simulink model "GNC2026W"  (R2024b)
settings: Solver=ode4  StartTime=0.0  StopTime=tsim  FixedStep=baseRate
values from neighbouring files (symbols this model uses):
  a = 1    [Run_Initializer.m]    (also in UKFoptimization.m)
  a1 = 0.236940    (= 0.23694)    [DrawARM.m]    (also in Run_Initializer.m = 2)
  a2 = 0.281536    [DrawARM.m]    (also in Run_Initializer.m = 2)
  a3 = 0.0621    [DrawARM.m]    (also in Run_Initializer.m = 2)
  A_c = eye(3)    [Run_Initializer.m]
  alpha = diag([a1; a2; a3])    [Run_Initializer.m]    (also in overlapping_trajectories.m = alpha_values1(ii); plotTrajectory.m = alpha_values(ii); plotfig.m = alpha_values(ii))
  b = 2    [Run_Initializer.m]    (also in UKFoptimization.m)
  b0 = 0.230400    (= 0.2304)    [DrawARM.m]
  b1 = 0.078980    (= 0.07898)    [DrawARM.m]
  b2 = 0.070384    [DrawARM.m]
  b3 = 0.070685    [DrawARM.m]
  CVrate = 1/5    (= 0.2)    [Run_Initializer.m]
  dt = baseRate    [Run_Initializer.m]    (also in UKFoptimization.m = 0.05; rms_plots.m = median(diff(tA)))
  F_u = zeros(3,1)    [Run_Initializer.m]
  fNum = 1    [Run_Initializer.m]
  gamma = r - (excess + shrink + bracketwidth)    (= 0.05023)    [DrawSpacecraft.m]    (also in Run_Initializer.m = diag([g1; g2; g3]))
  Gamma1_el = 0.12    [Run_Initializer.m]
  Gamma1_sh = 0.005    [Run_Initializer.m]
  Gamma1_wr = 0.025    [Run_Initializer.m]
  Gamma2_el = 5    [Run_Initializer.m]
  Gamma2_sh = 5    [Run_Initializer.m]
  Gamma2_wr = 5    [Run_Initializer.m]
  Gamma3_el = 10    [Run_Initializer.m]
  Gamma3_sh = 40    [Run_Initializer.m]
  Gamma3_wr = 40    [Run_Initializer.m]
  Gamma4_el = 0.039    [Run_Initializer.m]
  Gamma4_sh = 0.015    [Run_Initializer.m]
  Gamma4_wr = 0.029    [Run_Initializer.m]
  Gamma5_el = 800    [Run_Initializer.m]
  Gamma5_sh = 800    [Run_Initializer.m]
  Gamma5_wr = 800    [Run_Initializer.m]
  Gamma6_el = 0.000001    (= 1e-06)    [Run_Initializer.m]
  Gamma6_sh = 0.005    [Run_Initializer.m]
  Gamma6_wr = 0.02    [Run_Initializer.m]
  k = 5    [Run_Initializer.m]    (also in UKFoptimization.m)
  Kd_elarm = 0.8    [Run_Initializer.m]
  Kd_sharm = 1.0    (= 1)    [Run_Initializer.m]
  Kd_wrarm = 0.6    [Run_Initializer.m]
  Kp_elarm = 1.2    [Run_Initializer.m]
  Kp_sharm = 1.5    [Run_Initializer.m]
  Kp_wrarm = 1.0    (= 1)    [Run_Initializer.m]
  Mc_inv = inv(M_c)    [Run_Initializer.m]
  Phi = 73.2749*pi/180    (= 1.27888826407)    [DrawARM.m]
  PWMFreq = 5    [Run_Initializer.m]
  R = [cos(theta) -sin(theta) ... (first row only)    [Run_Initializer.m]    (also in UKFoptimization.m = diag([rx, rx, rt]))
  sep1 = 0.60    (= 0.6)    [Run_Initializer.m]
  sep2 = 0.30    (= 0.3)    [Run_Initializer.m]
  sep3 = 0.30    (= 0.3)    [Run_Initializer.m]
  Tz_lim_elarm = .1    (= 0.1)    [Run_Initializer.m]
  Tz_lim_sharm = .1    (= 0.1)    [Run_Initializer.m]
  Tz_lim_wrarm = .1    (= 0.1)    [Run_Initializer.m]
  VISinLoop = 1    [Run_Initializer.m]
  X1_blk = 0.4    [Run_Initializer.m]
  X2_blk = 0.4    [Run_Initializer.m]
  X3_blk = 0.4    [Run_Initializer.m]
  Y1_blk = 0.4    [Run_Initializer.m]
  Y2_blk = 0.4    [Run_Initializer.m]
  Y3_blk = 0.4    [Run_Initializer.m]
undefined symbols (not defined in the file or in its folder): baseRate, dataRate, DiscIntNeverNeededParam, drop_states_ARM, drop_states_BLACK, drop_states_BLUE, drop_states_RED, F_red_X_nominal, F_red_Y_nominal, F_thrusters_BLACK, F_thrusters_BLUE, F_thrusters_RED, home_states_BLACK, home_states_BLUE, home_states_RED, IBLACK, IBLUE, IDIST, IEE, init_states_BLACK, init_states_BLUE, init_states_RED, IPROX, IRED, K_BLACK, K_BLUE, K_RED, Kd_tb, Kd_tblue, Kd_tr, Kd_xb, Kd_xblue, Kd_xr, Kd_yb, Kd_yblue, Kd_yr, Kp_tb, Kp_tblue, Kp_tr, Kp_xb, Kp_xblue, Kp_xr, Kp_yb, Kp_yblue, Kp_yr, mBLACK, mBLUE, mDIST, mEE, mPROX, mRED, Phase0_End, Phase1_End, Phase2_End, Phase3_End, Phase3_SubPhase1_End, Phase3_SubPhase2_End, Phase3_SubPhase3_End, Phase3_SubPhase4_End, Phase4_End ... (+10)
libraries: simulink x30, nvidiaSharedBlocks x20, MainLibrary x5, dspinverses x3, commrandsrc3 x1, nvidiaIMUSensorslib x1
(part 3 of 9)

== system GNC2026W/3 - Control/Default PD (ARM) ==
  Action Port : ActionPort  ActionPortLabel=if(u1 == 1 )
  Constant7 : Constant
  Data Store Read2 : DataStoreRead  DataStoreName=ARM_Path  IndexOptions=Index vector (dialog)  Indices=1  OutputSizes=1
  Data Store Read4 : DataStoreRead  DataStoreName=isSim  IndexOptions=Index vector (dialog)  Indices=1  OutputSizes=1
  Data Store Write12 : DataStoreWrite  DataStoreName=ARM_Control_Mode  IndexOptions=Index vector (dialog)  Indices=1  OutputSizes=1
  Demux : Demux  Outputs=3
  "If 'simMode' set to '1', then this is a simulation and the dynamics will be simulated. Otherwise, this is an experiment, and the simulation will not be run." : If  IfExpression=u1 == 1
  Merge3 : Merge
  Merge4 : Merge
  Merge5 : Merge
  Mux : Mux  Inputs=3
  Passthrough for Experiment : Subsystem  TreatAsAtomicUnit=on
  Scope : Scope
  Simulated Position Controller : Subsystem  TreatAsAtomicUnit=on
  u : Outport
  wires:
  Passthrough for Experiment/3(q3_command) -> Merge5/2
  Data Store Read4/1 -> "If 'simMode' set to '1', then this is a simulation and the dynamics will be simulated. Otherwise, this is an experiment, and the simulation will not be run."/1
  Demux/3 -> Passthrough for Experiment/3(q3_desired), Simulated Position Controller/3(q3_desired)
  Simulated Position Controller/1(q1_command) -> Merge3/1
  Simulated Position Controller/3(q3_command) -> Merge5/1
  "If 'simMode' set to '1', then this is a simulation and the dynamics will be simulated. Otherwise, this is an experiment, and the simulation will not be run."/1 -> Simulated Position Controller/Action
  Demux/2 -> Passthrough for Experiment/2(q2_desired), Simulated Position Controller/2(q2_desired)
  Passthrough for Experiment/2(q2_command) -> Merge4/2
  Simulated Position Controller/2(q2_command) -> Merge4/1
  Constant7/1 -> Data Store Write12/1
  Passthrough for Experiment/1(q1_command) -> Merge3/2
  Demux/1 -> Passthrough for Experiment/1(q1_desired), Simulated Position Controller/1(q1_desired)
  "If 'simMode' set to '1', then this is a simulation and the dynamics will be simulated. Otherwise, this is an experiment, and the simulation will not be run."/2 -> Passthrough for Experiment/Action
  Merge3/1 -> Mux/1
  Merge4/1 -> Mux/2
  Merge5/1 -> Mux/3
  Mux/1 -> Scope/1, u/1
  Data Store Read2/1 -> Demux/1

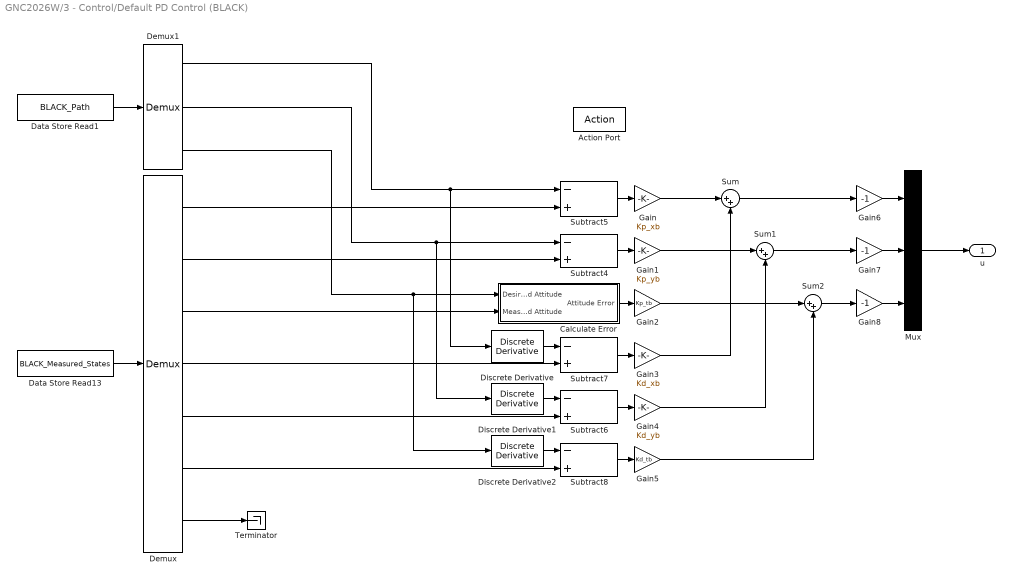
== system GNC2026W/3 - Control/Default PD Control (BLACK) ==
  Action Port : ActionPort  ActionPortLabel=if(u1 == 1 )
  Calculate Error : Subsystem
  Data Store Read1 : DataStoreRead  DataStoreName=BLACK_Path  IndexOptions=Index vector (dialog)  Indices=1  OutputSizes=1
  Data Store Read13 : DataStoreRead  DataStoreName=BLACK_Measured_States  IndexOptions=Index vector (dialog)  Indices=1  OutputSizes=1
  Demux : Demux  Outputs=[1,1,1,1,1,1,3]
  Demux1 : Demux  Outputs=3
  Discrete Derivative : simulink/Discrete/Discrete Derivative  gainval=1.0  ICPrevScaledInput=0.0  OutMin=[]  OutMax=[]  OutDataType=fixdt(1, 16)  OutScaling=2^-10  DoSatur=off
  Discrete Derivative1 : simulink/Discrete/Discrete Derivative  gainval=1.0  ICPrevScaledInput=0.0  OutMin=[]  OutMax=[]  OutDataType=fixdt(1, 16)  OutScaling=2^-10  DoSatur=off
  Discrete Derivative2 : simulink/Discrete/Discrete Derivative  gainval=1.0  ICPrevScaledInput=0.0  OutMin=[]  OutMax=[]  OutDataType=fixdt(1, 16)  OutScaling=2^-10  DoSatur=off
  Gain : Gain  Gain=Kp_xb
  Gain1 : Gain  Gain=Kp_yb
  Gain2 : Gain  Gain=Kp_tb
  Gain3 : Gain  Gain=Kd_xb
  Gain4 : Gain  Gain=Kd_yb
  Gain5 : Gain  Gain=Kd_tb
  Gain6 : Gain  Gain=-1
  Gain7 : Gain  Gain=-1
  Gain8 : Gain  Gain=-1
  Mux : Mux  Inputs=3
  Subtract{4..8} (5 alike) : Sum  Inputs=-+
  Sum : Sum  Inputs=|++
  Sum1 : Sum  Inputs=|++
  Sum2 : Sum  Inputs=|++
  Terminator : Terminator
  u : Outport
  wires:
  Demux/6 -> Subtract8/2
  Subtract8/1 -> Gain5/1
  Gain8/1 -> Mux/3
  Discrete Derivative2/1 -> Subtract8/1
  Gain1/1 -> Sum1/1
  Subtract5/1 -> Gain/1
  Discrete Derivative1/1 -> Subtract6/1
  Subtract6/1 -> Gain4/1
  Demux/2 -> Subtract4/2
  Demux/1 -> Subtract5/2
  Sum1/1 -> Gain7/1
  Demux/4 -> Subtract7/2
  Demux1/3 -> Calculate Error/1(Desired Attitude), Discrete Derivative2/1
  Sum/1 -> Gain6/1
  Subtract4/1 -> Gain1/1
  Demux/3 -> Calculate Error/2(Measured Attitude)
  Subtract7/1 -> Gain3/1
  Gain3/1 -> Sum/2
  Mux/1 -> u/1
  Gain4/1 -> Sum1/2
  Demux1/2 -> Discrete Derivative1/1, Subtract4/1
  Gain/1 -> Sum/1
  Demux/5 -> Subtract6/2
  Gain5/1 -> Sum2/2
  Discrete Derivative/1 -> Subtract7/1
  Demux1/1 -> Discrete Derivative/1, Subtract5/1
  Sum2/1 -> Gain8/1
  Calculate Error/1(Attitude Error) -> Gain2/1
  Gain7/1 -> Mux/2
  Gain6/1 -> Mux/1
  Gain2/1 -> Sum2/1
  Data Store Read13/1 -> Demux/1
  Demux/7 -> Terminator/1
  Data Store Read1/1 -> Demux1/1

== system GNC2026W/3 - Control/Default PD Control (BLUE) ==
  Action Port : ActionPort  ActionPortLabel=if(u1 == 1 )
  Calculate Error : Subsystem
  Data Store Read1 : DataStoreRead  DataStoreName=BLUE_Path  IndexOptions=Index vector (dialog)  Indices=1  OutputSizes=1
  Data Store Read2 : DataStoreRead  DataStoreName=BLUE_Measured_States  IndexOptions=Index vector (dialog)  Indices=1  OutputSizes=1
  Demux : Demux  Outputs=[1,1,1,1,1,1,3]
  Demux1 : Demux  Outputs=3
  Discrete Derivative : simulink/Discrete/Discrete Derivative  gainval=1.0  ICPrevScaledInput=0.0  OutMin=[]  OutMax=[]  OutDataType=fixdt(1, 16)  OutScaling=2^-10  DoSatur=off
  Discrete Derivative1 : simulink/Discrete/Discrete Derivative  gainval=1.0  ICPrevScaledInput=0.0  OutMin=[]  OutMax=[]  OutDataType=fixdt(1, 16)  OutScaling=2^-10  DoSatur=off
  Discrete Derivative2 : simulink/Discrete/Discrete Derivative  gainval=1.0  ICPrevScaledInput=0.0  OutMin=[]  OutMax=[]  OutDataType=fixdt(1, 16)  OutScaling=2^-10  DoSatur=off
  Gain : Gain  Gain=Kp_xblue
  Gain1 : Gain  Gain=Kp_yblue
  Gain2 : Gain  Gain=Kp_tblue
  Gain3 : Gain  Gain=Kd_xblue
  Gain4 : Gain  Gain=Kd_yblue
  Gain5 : Gain  Gain=Kd_tblue
  Gain6 : Gain  Gain=-1
  Gain7 : Gain  Gain=-1
  Gain8 : Gain  Gain=-1
  Mux3 : Mux  Inputs=3
  Subtract{4..8} (5 alike) : Sum  Inputs=-+
  Sum : Sum  Inputs=|++
  Sum1 : Sum  Inputs=|++
  Sum2 : Sum  Inputs=|++
  Terminator : Terminator
  u : Outport
  wires:
  Sum/1 -> Gain6/1
  Mux3/1 -> u/1
  Gain3/1 -> Sum/2
  Sum2/1 -> Gain8/1
  Gain5/1 -> Sum2/2
  Sum1/1 -> Gain7/1
  Gain6/1 -> Mux3/1
  Gain4/1 -> Sum1/2
  Gain1/1 -> Sum1/1
  Gain2/1 -> Sum2/1
  Gain8/1 -> Mux3/3
  Gain7/1 -> Mux3/2
  Gain/1 -> Sum/1
  Demux1/1 -> Discrete Derivative/1, Subtract5/1
  Discrete Derivative/1 -> Subtract7/1
  Demux1/3 -> Calculate Error/1(Desired Attitude), Discrete Derivative2/1
  Discrete Derivative1/1 -> Subtract6/1
  Demux/5 -> Subtract6/2
  Demux/3 -> Calculate Error/2(Measured Attitude)
  Demux/7 -> Terminator/1
  Data Store Read1/1 -> Demux1/1
  Demux/2 -> Subtract4/2
  Demux/1 -> Subtract5/2
  Demux/4 -> Subtract7/2
  Demux1/2 -> Discrete Derivative1/1, Subtract4/1
  Discrete Derivative2/1 -> Subtract8/1
  Data Store Read2/1 -> Demux/1
  Demux/6 -> Subtract8/2
  Subtract5/1 -> Gain/1
  Subtract4/1 -> Gain1/1
  Calculate Error/1(Attitude Error) -> Gain2/1
  Subtract7/1 -> Gain3/1
  Subtract6/1 -> Gain4/1
  Subtract8/1 -> Gain5/1

== system GNC2026W/3 - Control/Default PD Control (RED) ==
  Action Port : ActionPort  ActionPortLabel=if(u1 == 1 )
  Calculate Error : Subsystem
  Data Store Read1 : DataStoreRead  DataStoreName=RED_Path  IndexOptions=Index vector (dialog)  Indices=1  OutputSizes=1
  Data Store Read13 : DataStoreRead  DataStoreName=RED_Measured_States  IndexOptions=Index vector (dialog)  Indices=1  OutputSizes=1
  Demux : Demux  Outputs=[1,1,1,1,1,1,3]
  Demux1 : Demux  Outputs=3
  Discrete Derivative : simulink/Discrete/Discrete Derivative  gainval=1.0  ICPrevScaledInput=0.0  OutMin=[]  OutMax=[]  OutDataType=fixdt(1, 16)  OutScaling=2^-10  DoSatur=off
  Discrete Derivative1 : simulink/Discrete/Discrete Derivative  gainval=1.0  ICPrevScaledInput=0.0  OutMin=[]  OutMax=[]  OutDataType=fixdt(1, 16)  OutScaling=2^-10  DoSatur=off
  Discrete Derivative2 : simulink/Discrete/Discrete Derivative  gainval=1.0  ICPrevScaledInput=0.0  OutMin=[]  OutMax=[]  OutDataType=fixdt(1, 16)  OutScaling=2^-10  DoSatur=off
  Gain : Gain  Gain=Kp_xr
  Gain1 : Gain  Gain=Kp_yr
  Gain2 : Gain  Gain=Kp_tr
  Gain3 : Gain  Gain=Kd_xr
  Gain4 : Gain  Gain=Kd_yr
  Gain5 : Gain  Gain=Kd_tr
  Gain6 : Gain  Gain=-1
  Gain7 : Gain  Gain=-1
  Gain8 : Gain  Gain=-1
  Mux : Mux  Inputs=3
  Subtract{4..8} (5 alike) : Sum  Inputs=-+
  Sum : Sum  Inputs=|++
  Sum1 : Sum  Inputs=|++
  Sum2 : Sum  Inputs=|++
  Terminator : Terminator
  u1 : Outport
  wires:
  Gain6/1 -> Mux/1
  Gain8/1 -> Mux/3
  Gain1/1 -> Sum1/1
  Sum/1 -> Gain6/1
  Gain5/1 -> Sum2/2
  Gain3/1 -> Sum/2
  Sum1/1 -> Gain7/1
  Mux/1 -> u1/1
  Gain4/1 -> Sum1/2
  Sum2/1 -> Gain8/1
  Gain/1 -> Sum/1
  Gain7/1 -> Mux/2
  Gain2/1 -> Sum2/1
  Demux1/2 -> Discrete Derivative1/1, Subtract4/1
  Demux/2 -> Subtract4/2
  Demux1/3 -> Calculate Error/1(Desired Attitude), Discrete Derivative2/1
  Discrete Derivative1/1 -> Subtract6/1
  Demux/4 -> Subtract7/2
  Data Store Read13/1 -> Demux/1
  Demux/1 -> Subtract5/2
  Discrete Derivative/1 -> Subtract7/1
  Data Store Read1/1 -> Demux1/1
  Demux/5 -> Subtract6/2
  Demux/3 -> Calculate Error/2(Measured Attitude)
  Demux/7 -> Terminator/1
  Discrete Derivative2/1 -> Subtract8/1
  Demux1/1 -> Discrete Derivative/1, Subtract5/1
  Demux/6 -> Subtract8/2
  Subtract5/1 -> Gain/1
  Subtract4/1 -> Gain1/1
  Calculate Error/1(Attitude Error) -> Gain2/1
  Subtract7/1 -> Gain3/1
  Subtract6/1 -> Gain4/1
  Subtract8/1 -> Gain5/1

== system GNC2026W/3 - Control/Disable Control (ARM) ==
  Action Port : ActionPort  ActionPortLabel=else
  Constant7 : Constant  Value=0
  Data Store Write12 : DataStoreWrite  DataStoreName=ARM_Control_Mode  IndexOptions=Index vector (dialog)  Indices=1  OutputSizes=1
  Mux : Mux  Inputs=3
  Zero : Constant  Value=0  OutDataTypeStr=Inherit: Inherit via back propagation
  Out1 : Outport
  wires:
  Mux/1 -> Out1/1
  Zero/1 -> Mux/3, Mux/1, Mux/2
  Constant7/1 -> Data Store Write12/1

== system GNC2026W/3 - Control/Disable Thrusters (BLACK) ==
  Action Port : ActionPort  ActionPortLabel=else
  Mux : Mux  Inputs=3
  Zero : Constant  Value=0  OutDataTypeStr=Inherit: Inherit via back propagation
  Out1 : Outport
  wires:
  Zero/1 -> Mux/3, Mux/1, Mux/2
  Mux/1 -> Out1/1

== system GNC2026W/3 - Control/Disable Thrusters (BLUE) ==
  Action Port : ActionPort  ActionPortLabel=else
  Mux : Mux  Inputs=3
  Zero : Constant  Value=0  OutDataTypeStr=Inherit: Inherit via back propagation
  Out1 : Outport
  wires:
  Zero/1 -> Mux/3, Mux/1, Mux/2
  Mux/1 -> Out1/1

== system GNC2026W/3 - Control/Disable Thrusters (RED) ==
  Action Port : ActionPort  ActionPortLabel=else
  Mux : Mux  Inputs=3
  Zero : Constant  Value=0  OutDataTypeStr=Inherit: Inherit via back propagation
  u : Outport
  wires:
  Zero/1 -> Mux/3, Mux/1, Mux/2
  Mux/1 -> u/1

== system GNC2026W/Check Connection/Change BLACK Behavior ==
  Action Port : ActionPort  ActionPortLabel=if(u1 == 2 & u2 == 0)
  Constant1 : Constant  OutDataTypeStr=int32
  UDP Send : nvidiaSharedBlocks/UDP Send  remoteURL='255.255.255.255'  remotePort=33002  localURL='0.0.0.0'  localPortSource=Automatically determine  localPort=-1  sampletime=-1  blockPlatform=NVIDIA  separateLengthPort=0
      settings: LibrarySourceBlock=nvidiaNetworklib/UDP Send
  wires:
  Constant1/1 -> UDP Send/1

== system GNC2026W/Check Connection/Change BLUE Behavior ==
  Action Port : ActionPort  ActionPortLabel=if(u1 == 3 & u2 == 0)
  Constant1 : Constant  OutDataTypeStr=int32
  UDP Send : nvidiaSharedBlocks/UDP Send  remoteURL='255.255.255.255'  remotePort=33003  localURL='0.0.0.0'  localPortSource=Automatically determine  localPort=-1  sampletime=-1  blockPlatform=NVIDIA  separateLengthPort=0
      settings: LibrarySourceBlock=nvidiaNetworklib/UDP Send
  wires:
  Constant1/1 -> UDP Send/1

== system GNC2026W/Check Connection/Change RED Behavior ==
  Action Port : ActionPort  ActionPortLabel=if(u1 == 1 & u2 == 0)
  Constant1 : Constant  OutDataTypeStr=int32
  UDP Send : nvidiaSharedBlocks/UDP Send  remoteURL='255.255.255.255'  remotePort=33001  localURL='0.0.0.0'  localPortSource=Automatically determine  localPort=-1  sampletime=-1  blockPlatform=NVIDIA  separateLengthPort=0
      settings: LibrarySourceBlock=nvidiaNetworklib/UDP Send
  wires:
  Constant1/1 -> UDP Send/1

== system GNC2026W/Data Logger Subsystem/Separation ==
  Data Store Read31 : DataStoreRead  DataStoreName=RED_Measured_States  IndexOptions=Index vector (dialog)  Indices=1  OutputSizes=1
  Data Store Read32 : DataStoreRead  DataStoreName=BLACK_Measured_States  IndexOptions=Index vector (dialog)  Indices=1  OutputSizes=1
  MATLAB Function : MATLAB Function  TreatAsAtomicUnit=on
  L : Outport
  wires:
  MATLAB Function/1(L) -> L/1
  Data Store Read32/1 -> MATLAB Function/2(BLACK_path)
  Data Store Read31/1 -> MATLAB Function/1(RED_path)

== system GNC2026W/Debugger/Change BLACK Behavior ==
  Action Port : ActionPort  ActionPortLabel=if(u1 == 2 & u2 == 0)
  Data Store Read2 : DataStoreRead  DataStoreName=BLACK_Logger  IndexOptions=Index vector (dialog)  Indices=1  OutputSizes=1
  Data Type Conversion1 : DataTypeConversion  OutDataTypeStr=uint8  SaturateOnIntegerOverflow=off  RndMeth=Floor
  String to ASCII1 : StringToASCII
  UDP Send1 : nvidiaSharedBlocks/UDP Send  remoteURL='255.255.255.255'  remotePort=55000  localURL='0.0.0.0'  localPortSource=Automatically determine  localPort=-1  sampletime=-1  blockPlatform=NVIDIA  separateLengthPort=0
      settings: LibrarySourceBlock=nvidiaNetworklib/UDP Send
  wires:
  Data Type Conversion1/1 -> UDP Send1/1
  Data Store Read2/1 -> String to ASCII1/1
  String to ASCII1/1 -> Data Type Conversion1/1

== system GNC2026W/Debugger/Change BLUE Behavior ==
  Action Port : ActionPort  ActionPortLabel=if(u1 == 3 & u2 == 0)
  Data Store Read : DataStoreRead  DataStoreName=BLUE_Logger  IndexOptions=Index vector (dialog)  Indices=1  OutputSizes=1
  Data Type Conversion2 : DataTypeConversion  OutDataTypeStr=uint8  SaturateOnIntegerOverflow=off  RndMeth=Floor
  String to ASCII2 : StringToASCII
  UDP Send2 : nvidiaSharedBlocks/UDP Send  remoteURL='255.255.255.255'  remotePort=55000  localURL='0.0.0.0'  localPortSource=Automatically determine  localPort=-1  sampletime=-1  blockPlatform=NVIDIA  separateLengthPort=0
      settings: LibrarySourceBlock=nvidiaNetworklib/UDP Send
  wires:
  Data Type Conversion2/1 -> UDP Send2/1
  String to ASCII2/1 -> Data Type Conversion2/1
  Data Store Read/1 -> String to ASCII2/1

== system GNC2026W/Debugger/Change RED Behavior ==
  Action Port : ActionPort  ActionPortLabel=if(u1 == 1 & u2 == 0)
  Data Store Read : DataStoreRead  DataStoreName=RED_Logger  IndexOptions=Index vector (dialog)  Indices=1  OutputSizes=1
  Data Type Conversion : DataTypeConversion  OutDataTypeStr=uint8  SaturateOnIntegerOverflow=off  RndMeth=Floor
  String to ASCII : StringToASCII
  UDP Send3 : nvidiaSharedBlocks/UDP Send  remoteURL='255.255.255.255'  remotePort=55000  localURL='0.0.0.0'  localPortSource=Automatically determine  localPort=-1  sampletime=-1  blockPlatform=NVIDIA  separateLengthPort=0
      settings: LibrarySourceBlock=nvidiaNetworklib/UDP Send
  wires:
  Data Store Read/1 -> String to ASCII/1
  Data Type Conversion/1 -> UDP Send3/1
  String to ASCII/1 -> Data Type Conversion/1

== system GNC2026W/Float Code/Enable Pucks ==
  Action Port : ActionPort  ActionPortLabel=if(u1 == 0)
  Data Store Read1 : DataStoreRead  DataStoreName=Float_State  IndexOptions=Index vector (dialog)  Indices=1  OutputSizes=1
  GPIO Write1 : MainLibrary/Jetson Functions/GPIO Write  gpioPin=428  pinDirection=1
      settings: SourceProductName=SPOT Custom Library
  wires:
  Data Store Read1/1 -> GPIO Write1/1

== system GNC2026W/Gyro.//Accel. Code/Log Gyro//Accel ==
  Action Port : ActionPort  ActionPortLabel=if(u1 == 0)
  Data Store Read : DataStoreRead  DataStoreName=WhoAmI  IndexOptions=Index vector (dialog)  Indices=1  OutputSizes=1
  Data Store Write10 : DataStoreWrite  DataStoreName=BLACK_IMU_Measurements  IndexOptions=Index vector (dialog)  Indices=1  OutputSizes=1
  Data Store Write11 : DataStoreWrite  DataStoreName=BLUE_IMU_Measurements  IndexOptions=Index vector (dialog)  Indices=1  OutputSizes=1
  Data Store Write9 : DataStoreWrite  DataStoreName=RED_IMU_Measurements  IndexOptions=Index vector (dialog)  Indices=1  OutputSizes=1
  Demux : Demux  Outputs=3
  Demux1 : Demux  Outputs=3
  Gyroscope/Accelerometer : nvidiaIMUSensorslib/BMI160  I2CModule=1  I2CAddress=0x69  EnableSecondaryMag=on  MagnetometerI2CAddress=0x10  BitRate=1000000  IsActiveAccel=on  IsActiveGyro=on  IsActiveMag=off  IsActiveTemperature=off  IsIntSource=off  IsTapEventSource=off  IsHighGEventSource=off  IsAnyMotionEventSource=off  IsAccelStatus=off  IsGyroStatus=off  IsMagStatus=off  AccelerationRange=+/- 2g  AccelerometerODR=100 Hz  IsEnableAccelLowPassFilter=off  AccelerometerFilterMode=Normal  GyroscopeRange=125 dps  GyroscopeODR=100 Hz  IsEnableGyroLowPassFilter=off  GyroscopeFilterMode=Normal  MagnetometerODR=25 Hz  IsSingleTap=off  SingleTapQuietTimeThreshold=30 ms  SingleTapShockTimeThreshold=50 ms  SingleTapAmplitudeThreshold2g=0.1  SingleTapAmplitudeThreshold4g=0.1  SingleTapAmplitudeThreshold8g=0.2  SingleTapAmplitudeThreshold16g=0.3  InterruptPinSingleTap=INT1  IsDoubleTap=off  DoubleTapDurationTimeThreshold=50 ms  InterruptPinDoubleTap=INT1  IsHighGDetection=off  HighGTimeThreshold=2.5  HighGAmplitudeThreshold2g=0.1  HighGAmplitudeThreshold4g=0.1  HighGAmplitudeThreshold8g=0.1  HighGAmplitudeThreshold16g=0.1  InterruptPinHighG=INT1  IsAnyMotion=off  AnyMotionTimeThreshold=1  AnyMotionAmplitudeThreshold2g=0.1  AnyMotionAmplitudeThreshold4g=0.1  AnyMotionAmplitudeThreshold8g=0.1  AnyMotionAmplitudeThreshold16g=0.1  InterruptPinAnyMotion=INT1  IsSlowMotion=off  SlowMotionTimeThreshold=1  SlowMotionAmplitudeThreshold2g=0.1  SlowMotionAmplitudeThreshold4g=0.1  SlowMotionAmplitudeThreshold8g=0.1  SlowMotionAmplitudeThreshold16g=0.1  InterruptPinSlowMotion=INT1  IsFlatDetection=off  FlatThetaThreshold=5  FlatTimeThreshold=640 ms  InterruptPinFlat=INT1  IsDataReady=off  InterruptPinDataReady=INT1  IsFifo=off  FifoMode=Full Buffer  InterruptPinFifo=INT1  DataType=double  SampleTime=-1
  Mux : Mux  Inputs=3
  Mux1 : Mux  Inputs=3
  Mux2 : Mux  Inputs=3
  Parse IMU Data : MATLAB Function  TreatAsAtomicUnit=on
  Terminator : Terminator
  Terminator1 : Terminator
  Terminator2 : Terminator
  wires:
  Demux1/3 -> Parse IMU Data/4(IMU_Gz)
  Gyroscope/Accelerometer/1 -> Demux/1
  Demux1/1 -> Terminator1/1
  Parse IMU Data/4(BLACK_IMU_Ax) -> Mux1/1
  Parse IMU Data/1(RED_IMU_Ax) -> Mux/1
  Parse IMU Data/8(BLUE_IMU_Ay) -> Mux2/2
  Parse IMU Data/3(RED_IMU_Gz) -> Mux/3
  Demux/3 -> Terminator/1
  Parse IMU Data/6(BLACK_IMU_Gz) -> Mux1/3
  Parse IMU Data/5(BLACK_IMU_Ay) -> Mux1/2
  Demux1/2 -> Terminator2/1
  Parse IMU Data/9(BLUE_IMU_Gz) -> Mux2/3
  Gyroscope/Accelerometer/2 -> Demux1/1
  Parse IMU Data/2(RED_IMU_Ay) -> Mux/2
  Parse IMU Data/7(BLUE_IMU_Ax) -> Mux2/1
  Demux/2 -> Parse IMU Data/3(IMU_Ay)
  Data Store Read/1 -> Parse IMU Data/1(WhoAmI)
  Demux/1 -> Parse IMU Data/2(IMU_Ax)
  Mux/1 -> Data Store Write9/1
  Mux1/1 -> Data Store Write10/1
  Mux2/1 -> Data Store Write11/1

== system GNC2026W/Manipulator Encoder Data/Change ARM Behavior ==
  Action Port : ActionPort  ActionPortLabel=if(u1 == 1 & u2 == 0)
  Data Store Write : DataStoreWrite  DataStoreName=ARM_Measured_States  IndexOptions=Index vector (dialog)  Indices=1  OutputSizes=1
  Delay : Delay  DelayLength=1
  Delay1 : Delay  DelayLength=1
  Delay2 : Delay  DelayLength=1
  Mux : Mux  Inputs=6
  Read Joint Positions using Dynamixel Encoders : MainLibrary/Dynamixel Functions/Read Joint Positions using  Dynamixel Encoders  SampleTime=baseRate
      settings: SourceProductName=SPOT Custom Library
  wires:
  Delay/1 -> Read Joint Positions using Dynamixel Encoders/1
  Read Joint Positions using Dynamixel Encoders/5 -> Mux/5
  Read Joint Positions using Dynamixel Encoders/6 -> Mux/6
  Delay1/1 -> Read Joint Positions using Dynamixel Encoders/2
  Read Joint Positions using Dynamixel Encoders/2 -> Mux/2, Delay1/1
  Delay2/1 -> Read Joint Positions using Dynamixel Encoders/3
  Read Joint Positions using Dynamixel Encoders/1 -> Mux/1, Delay/1
  Read Joint Positions using Dynamixel Encoders/3 -> Mux/3, Delay2/1
  Read Joint Positions using Dynamixel Encoders/4 -> Mux/4
  Mux/1 -> Data Store Write/1

== system GNC2026W/Navigation Filter/If Action Subsystem ==
  Action Port : ActionPort  ActionPortLabel=if(u1 >= u2)
  Constant : Constant  Value=fNum
  Data Store Write2 : DataStoreWrite  DataStoreName=BLACK_Filtered_States  IndexOptions=Index vector (dialog)  Indices=1  OutputSizes=1
  EKF : Subsystem  TreatAsAtomicUnit=on
  If : If  IfExpression=u1 == 1  ElseIfExpressions=u1 == 2, u1 == 3  ShowElse=off
  MEKF : Subsystem  TreatAsAtomicUnit=on
  Merge : Merge  Inputs=3
  Scope1 : Scope
  UKF : Subsystem  TreatAsAtomicUnit=on
  wires:
  Merge/1 -> Data Store Write2/1, Scope1/1
  EKF/1(BLKest) -> Merge/3
  MEKF/1(BLKest) -> Merge/2
  If/2 -> MEKF/Action
  If/1 -> UKF/Action
  Constant/1 -> If/1
  UKF/1(BLKest) -> Merge/1
  If/3 -> EKF/Action

== system GNC2026W/PhaseSpace Camera Code/Initialize Universal Time (Simulation) ==
  Action Port : ActionPort  ActionPortLabel=elseif(u1 == 1)
  Set Universal Time (If this is a simulation) : Clock
  Universal_Time : DataStoreWrite  DataStoreName=Univ_Time  IndexOptions=Index vector (dialog)  Indices=1  OutputSizes=1
  wires:
  Set Universal Time (If this is a simulation)/1 -> Universal_Time/1

== system GNC2026W/PhaseSpace Camera Code/Use Hardware to Obtain States ==
  Action Port : ActionPort  ActionPortLabel=if(u1 == 0)
  Demux : Demux  Outputs=[4,3,3,9]
  Demux1 : Demux  Outputs=[3,3,3]
  Receive and Process Phasespace Data : Subsystem
  Store BLACK Data : Subsystem
  Store BLUE Data : Subsystem
  Store RED Data : Subsystem
  wires:
  Receive and Process Phasespace Data/1(PhaseSpace Data) -> Demux/1
  Demux/1 -> Store RED Data/1(RED Data)
  Demux/2 -> Store BLACK Data/1(BLACK Data)
  Demux/3 -> Store BLUE Data/1(BLUE Data)
  Demux/4 -> Demux1/1
  Demux1/1 -> Store RED Data/2(RED Velocities)
  Demux1/2 -> Store BLACK Data/2(BLACK Velocities)
  Demux1/3 -> Store BLUE Data/2(BLUE Velocities)
  Receive and Process Phasespace Data/2(PhaseSpace Clock) -> Store RED Data/3(PS Clock), Store BLACK Data/3(PS Clock), Store BLUE Data/3(PS Clock)

== system GNC2026W/Platform Identification/Subsystem ==
  Action Port : ActionPort  ActionPortLabel=if(u1 == 0)
  Data Store Write : DataStoreWrite  DataStoreName=WhoAmI  IndexOptions=Index vector (dialog)  Indices=1  OutputSizes=1
  WhoAmI : MainLibrary/WhoAmI  SampleTime=baseRate
      settings: SourceProductName=SPOT Custom Library
  wires:
  WhoAmI/1 -> Data Store Write/1

== system GNC2026W/Receive CV Data/CV UDP ==
  Action Port : ActionPort  ActionPortLabel=if(u1 == 0)
  Cast To Double{,1..3} (4 alike) : DataTypeConversion  OutDataTypeStr=double  SaturateOnIntegerOverflow=off  RndMeth=Floor
  Constant : Constant  Value=VISinLoop
  Data Store Write : DataStoreWrite  DataStoreName=VIS_LAR_States  IndexOptions=Index vector (dialog)  Indices=1  OutputSizes=1
  Demux : Demux
  Gain : Gain  Gain=-1
  If : If  IfExpression=u1 == 1  ShowElse=off
  Mux : Mux  Inputs=3
  Reading isValid : Subsystem  TreatAsAtomicUnit=on
  Terminator : Terminator
  UDP Receive : nvidiaSharedBlocks/UDP Receive  localURL='0.0.0.0'  localPort=50005  remoteURL='0.0.0.0'  remotePort=-1  recvBufferSize=8192  signalDatatype=single  dims=4  isVarSize=off  showBlockingTime=off  blockingTime=0  sampletime=baseRate  blockPlatform=NVIDIA
      settings: LibrarySourceBlock=nvidiaNetworklib/UDP Receive
  wires:
  UDP Receive/2 -> Terminator/1
  UDP Receive/1 -> Demux/1
  Demux/2 -> Cast To Double/1
  Demux/3 -> Cast To Double1/1
  Demux/4 -> Cast To Double2/1
  Cast To Double/1 -> Mux/1
  Cast To Double1/1 -> Gain/1
  Demux/1 -> Cast To Double3/1
  Cast To Double3/1 -> Reading isValid/1(In1)
  Mux/1 -> Data Store Write/1
  Gain/1 -> Mux/2
  Cast To Double2/1 -> Mux/3
  If/1 -> Reading isValid/Action
  Constant/1 -> If/1

== system GNC2026W/Receive Data from Orin/Subsystem ==
  Action Port : ActionPort  ActionPortLabel=if(u1 == 0)
  Cast To Double{,1..3} (4 alike) : DataTypeConversion  OutDataTypeStr=double  SaturateOnIntegerOverflow=off  RndMeth=Floor
  Data Store Write : DataStoreWrite  DataStoreName=VIS_Measured_States  IndexOptions=Index vector (dialog)  Indices=1  OutputSizes=1
  Data Store Write1 : DataStoreWrite  DataStoreName=VIS_Confidence  IndexOptions=Index vector (dialog)  Indices=1  OutputSizes=1
  Demux : Demux
  Mux : Mux  Inputs=3
  Terminator : Terminator
  UDP Receive : nvidiaSharedBlocks/UDP Receive  localURL='0.0.0.0'  localPort=36845  remoteURL='0.0.0.0'  remotePort=-1  recvBufferSize=8192  signalDatatype=single  dims=4  isVarSize=off  showBlockingTime=off  blockingTime=0  sampletime=baseRate  blockPlatform=NVIDIA
      settings: LibrarySourceBlock=nvidiaNetworklib/UDP Receive
  wires:
  UDP Receive/2 -> Terminator/1
  UDP Receive/1 -> Demux/1
  Demux/1 -> Cast To Double/1
  Demux/2 -> Cast To Double1/1
  Demux/3 -> Cast To Double2/1
  Demux/4 -> Cast To Double3/1
  Cast To Double/1 -> Mux/1
  Cast To Double1/1 -> Mux/2
  Cast To Double2/1 -> Mux/3
  Mux/1 -> Data Store Write/1
  Cast To Double3/1 -> Data Store Write1/1

== system GNC2026W/Robotic Arm Code/Change ARM Behavior ==
  Action Port : ActionPort  ActionPortLabel=if(u1 == 1 & u2 == 0)
  Arm Control Mode : DataStoreRead  DataStoreName=ARM_Control_Mode  IndexOptions=Index vector (dialog)  Indices=1  OutputSizes=1
  Command : DataStoreRead  DataStoreName=ARM_Controls  IndexOptions=Index vector (dialog)  Indices=1  OutputSizes=1
  "Control Dynamixel Actuators in either Position, Current, or Speed Control Modes" : MainLibrary/Dynamixel Functions/Control Dynamixel Actuators in  either Position, Current, or Speed  Control Modes  POSITION_P_GAIN=400  POSITION_I_GAIN=0  POSITION_D_GAIN=200  MAX_POSITION=3072  MIN_POSITION=1024  MOVE_TIME=0  CURRENT_LIMIT=850  SPEED_P_GAIN=400  SPEED_I_GAIN=100  VELOCITY_LIMIT=20  ACCELERATION_TIME=0  SampleTime=baseRate
      settings: SourceProductName=SPOT Custom Library
  Demux : Demux  Outputs=3
  wires:
  Arm Control Mode/1 -> "Control Dynamixel Actuators in either Position, Current, or Speed Control Modes"/1
  Command/1 -> Demux/1
  Demux/1 -> "Control Dynamixel Actuators in either Position, Current, or Speed Control Modes"/2
  Demux/2 -> "Control Dynamixel Actuators in either Position, Current, or Speed Control Modes"/3
  Demux/3 -> "Control Dynamixel Actuators in either Position, Current, or Speed Control Modes"/4

== system GNC2026W/Send Data to Orin/Subsystem ==
  Action Port : ActionPort  ActionPortLabel=if(u1 == 0)
  BLACK States : DataStoreRead  DataStoreName=BLACK_Measured_States  IndexOptions=Index vector (dialog)  Indices=1  OutputSizes=1
  BLUE States : DataStoreRead  DataStoreName=BLUE_Measured_States  IndexOptions=Index vector (dialog)  Indices=1  OutputSizes=1
  Mux : Mux
  RED States : DataStoreRead  DataStoreName=RED_Measured_States  IndexOptions=Index vector (dialog)  Indices=1  OutputSizes=1
  Time : DataStoreRead  DataStoreName=Univ_Time  IndexOptions=Index vector (dialog)  Indices=1  OutputSizes=1
  UDP Send : nvidiaSharedBlocks/UDP Send  remoteURL='192.168.1.115'  remotePort=46875  localURL='0.0.0.0'  localPortSource=Automatically determine  localPort=-1  sampletime=-1  blockPlatform=NVIDIA  separateLengthPort=0
      settings: LibrarySourceBlock=nvidiaNetworklib/UDP Send
  wires:
  Mux/1 -> UDP Send/1
  Time/1 -> Mux/1
  RED States/1 -> Mux/2
  BLACK States/1 -> Mux/3
  BLUE States/1 -> Mux/4

== system GNC2026W/Simulate Plant Dynamics/BLACK Dynamics ==
  Add Noise : RandomNumber  Variance=1e-9  SampleTime=baseRate
  Calculated & Store Measured States : Subsystem
  Calculated & Store True States : Subsystem
  Data @ Measurement Rate : Subsystem
  Dynamics Model for BLACK : Subsystem  SystemSampleTime=serverRate
      settings: PortSchema="{\"entries\":[{\"content\":{\"sides\":[{\"content\":{\"connectorIds\":[\"In1\"]},\"type\":\"ConnectorPlacement.EquallySpacedRectSide\",\"uuid\":\"9df3cfb7-f920-4c45-b004-2d63eab5f007\"},{\"content\":{\"side\":\"RIGHT\"},\"type\":\"ConnectorPlacement.EquallySpacedRectSide\",\"uuid\":\"24f4b70f-864f-4cab-bc2b-b450467a01b3\"},{\"content\":{\"connectorIds\":[\"Out1\"],\"side\":\"TOP\"},\"type\":\"ConnectorPlacement.EquallySpacedRectSide\",\"uuid\":\"64c0236c-f70a-4099-950e-ee3e8643e7f2\"}]},\"type\":\"ConnectorPlacement.EquallySpacedConnector\",\"uuid\":\"dd7c693a-185b-4c5f-873e-b9df56bea395\"}],\"packageUris\":[\"http://schema.mathworks.com/mf0/Connector/R2020b\"],\"version\":\"1.0\"}"
  Saturated Control Commands for BLACK : DataStoreRead  DataStoreName=BLACK_Saturated_Controls  IndexOptions=Index vector (dialog)  Indices=1  OutputSizes=1
  "Simulated Noise " : Subsystem
  Sum : Sum  Inputs=++|
  wires:
  Dynamics Model for BLACK/1(states) -> Sum/2, Calculated & Store True States/1(y)
  Data @ Measurement Rate/2(Time Step) -> Calculated & Store Measured States/2(dt)
  Saturated Control Commands for BLACK/1 -> Dynamics Model for BLACK/1(control_inputs)
  Data @ Measurement Rate/1(Data Held) -> "Simulated Noise "/1(true states), Calculated & Store Measured States/1(y)
  Sum/1 -> Data @ Measurement Rate/1(Data Input)
  Add Noise/1 -> Sum/1

== system GNC2026W/Simulate Plant Dynamics/BLUE Dynamics ==
  Add Noise : RandomNumber  Variance=1e-9  SampleTime=baseRate
  BLUE  Dynamics Model : Subsystem  SystemSampleTime=serverRate
      settings: PortSchema="{\"entries\":[{\"content\":{\"sides\":[{\"content\":{\"connectorIds\":[\"In1\"]},\"type\":\"ConnectorPlacement.EquallySpacedRectSide\",\"uuid\":\"9df3cfb7-f920-4c45-b004-2d63eab5f007\"},{\"content\":{\"side\":\"RIGHT\"},\"type\":\"ConnectorPlacement.EquallySpacedRectSide\",\"uuid\":\"24f4b70f-864f-4cab-bc2b-b450467a01b3\"},{\"content\":{\"connectorIds\":[\"Out1\"],\"side\":\"TOP\"},\"type\":\"ConnectorPlacement.EquallySpacedRectSide\",\"uuid\":\"64c0236c-f70a-4099-950e-ee3e8643e7f2\"}]},\"type\":\"ConnectorPlacement.EquallySpacedConnector\",\"uuid\":\"dd7c693a-185b-4c5f-873e-b9df56bea395\"}],\"packageUris\":[\"http://schema.mathworks.com/mf0/Connector/R2020b\"],\"version\":\"1.0\"}"
  Calculated & Store Measured States : Subsystem
  Calculated & Store True States : Subsystem
  Data @ Measurement Rate : Subsystem
  Saturated Control Commands for BLUE : DataStoreRead  DataStoreName=BLUE_Saturated_Controls  IndexOptions=Index vector (dialog)  Indices=1  OutputSizes=1
  Sum1 : Sum  Inputs=++|
  wires:
  Saturated Control Commands for BLUE/1 -> BLUE  Dynamics Model/1(control_inputs)
  Data @ Measurement Rate/2(Time Step) -> Calculated & Store Measured States/2(dt)
  Add Noise/1 -> Sum1/1
  BLUE  Dynamics Model/1(states) -> Sum1/2, Calculated & Store True States/1(y)
  Sum1/1 -> Data @ Measurement Rate/1(Data Input)
  Data @ Measurement Rate/1(Data Held) -> Calculated & Store Measured States/1(y)

== system GNC2026W/Simulate Plant Dynamics/RED and ARM Dynamics ==
  Constant : Constant  Value=platformSelection
  If : If  IfExpression=u1 == 4 | u1 == 5 | u1 == 10 | u1 == 11
  RED + ARM : Subsystem  TreatAsAtomicUnit=on
  RED Only : Subsystem  TreatAsAtomicUnit=on
  wires:
  If/1 -> RED + ARM/Action
  Constant/1 -> If/1
  If/2 -> RED Only/Action

== system GNC2026W/Thruster Control Code/Change BLACK Behavior ==
  note: Calculate the percentage of time each thruster must be on, and send to the PWM blocks.
  note: Using the attitude, rotate the forces into the body frame.
  note: Calculate which thrusters must be turned on and for how long.
  Action Port : ActionPort  ActionPortLabel=if(u1 == 2 | u2 == 1)
  BLACK Controls : DataStoreRead  DataStoreName=BLACK_Controls  IndexOptions=Index vector (dialog)  Indices=1  OutputSizes=1
  BLACK States : DataStoreRead  DataStoreName=BLACK_Measured_States  IndexOptions=Index vector (dialog)  Indices=1  OutputSizes=1
  Calculate Duty Cycle : Subsystem
  Data Store Write2 : DataStoreWrite  DataStoreName=BLACK_Saturated_Controls  IndexOptions=Index vector (dialog)  Indices=1  OutputSizes=1
  Demux1 : Demux  Outputs=[2,1]
  Demux2 : Demux  Outputs=[2,1,6]
  Mux : Mux  Inputs=2
  Rotate Forces to Body : Subsystem
  Terminator : Terminator
  Terminator1 : Terminator
  BLACK DC : Outport  VectorParamsAs1DForOutWhenUnconnected=off
  wires:
  Calculate Duty Cycle/2(Saturated Forces Moments) -> Data Store Write2/1
  Rotate Forces to Body/1(F_b) -> Mux/1
  Demux1/2 -> Mux/2
  Calculate Duty Cycle/1(Duty Cycle) -> BLACK DC/1
  Mux/1 -> Calculate Duty Cycle/1("[Fx_b; Fy_b; Tz]")
  BLACK Controls/1 -> Demux1/1
  Demux1/1 -> Rotate Forces to Body/1("F_I ")
  BLACK States/1 -> Demux2/1
  Demux2/1 -> Terminator/1
  Demux2/3 -> Terminator1/1
  Demux2/2 -> Calculate Duty Cycle/2(Measured Attitude), Rotate Forces to Body/2(Rz)

== system GNC2026W/Thruster Control Code/Change BLUE Behavior ==
  note: Calculate the percentage of time each thruster must be on, and send to the PWM blocks.
  note: Using the attitude, rotate the forces into the body frame.
  note: Calculate which thrusters must be turned on and for how long.
  Action Port : ActionPort  ActionPortLabel=if(u1 == 3 | u2 == 1)
  Calculate Duty Cycle : Subsystem
  Data Store Read : DataStoreRead  DataStoreName=BLUE_Controls  IndexOptions=Index vector (dialog)  Indices=1  OutputSizes=1
  Data Store Read1 : DataStoreRead  DataStoreName=BLUE_Measured_States  IndexOptions=Index vector (dialog)  Indices=1  OutputSizes=1
  Data Store Write3 : DataStoreWrite  DataStoreName=BLUE_Saturated_Controls  IndexOptions=Index vector (dialog)  Indices=1  OutputSizes=1
  Demux : Demux  Outputs=[2,1]
  Demux1 : Demux  Outputs=[2,1,6]
  Mux1 : Mux  Inputs=2
  Rotate Forces to Body : Subsystem
  Terminator : Terminator
  Terminator1 : Terminator
  BLUE DC : Outport  VectorParamsAs1DForOutWhenUnconnected=off
  wires:
  Calculate Duty Cycle/1(Duty Cycle) -> BLUE DC/1
  Rotate Forces to Body/1(F_b) -> Mux1/1
  Demux/2 -> Mux1/2
  Mux1/1 -> Calculate Duty Cycle/1("[Fx_b; Fy_b; Tz]")
  Calculate Duty Cycle/2(Saturated Forces Moments) -> Data Store Write3/1
  Data Store Read/1 -> Demux/1
  Demux/1 -> Rotate Forces to Body/1("F_I ")
  Data Store Read1/1 -> Demux1/1
  Demux1/2 -> Calculate Duty Cycle/2(Measured Attitude), Rotate Forces to Body/2(Rz)
  Demux1/1 -> Terminator/1
  Demux1/3 -> Terminator1/1

== system GNC2026W/Thruster Control Code/Change RED Behavior ==
  note: Calculate which thrusters must be turned on and for how long.
  note: Calculate the percentage of time each thruster must be on, and send to the PWM blocks.
  note: Using the attitude, rotate the forces into the body frame.
  Action Port : ActionPort  ActionPortLabel=if(u1 == 1 | u2 == 1)
  Calculate Duty Cycle : Subsystem
  Data Store Read : DataStoreRead  DataStoreName=RED_Controls  IndexOptions=Index vector (dialog)  Indices=1  OutputSizes=1
  Data Store Read1 : DataStoreRead  DataStoreName=RED_Measured_States  IndexOptions=Index vector (dialog)  Indices=1  OutputSizes=1
  Data Store Write1 : DataStoreWrite  DataStoreName=RED_Saturated_Controls  IndexOptions=Index vector (dialog)  Indices=1  OutputSizes=1
  Demux : Demux  Outputs=[2,1]
  Demux1 : Demux  Outputs=[2,1,6]
  Mux1 : Mux  Inputs=2
  Rotate Forces to Body : Subsystem
  Terminator : Terminator
  Terminator1 : Terminator
  RED DC : Outport  VectorParamsAs1DForOutWhenUnconnected=off
  wires:
  Demux/1 -> Rotate Forces to Body/1("F_I ")
  Mux1/1 -> Calculate Duty Cycle/1("[Fx_b; Fy_b; Tz]")
  Demux/2 -> Mux1/2
  Demux1/2 -> Calculate Duty Cycle/2(Measured Attitude), Rotate Forces to Body/2(Rz)
  Rotate Forces to Body/1(F_b) -> Mux1/1
  Data Store Read/1 -> Demux/1
  Demux1/1 -> Terminator/1
  Demux1/3 -> Terminator1/1
  Data Store Read1/1 -> Demux1/1
  Calculate Duty Cycle/2(Saturated Forces Moments) -> Data Store Write1/1
  Calculate Duty Cycle/1(Duty Cycle) -> RED DC/1

== system GNC2026W/Time Sync./Change BLACK Behavior ==
  Action Port : ActionPort  ActionPortLabel=if(u1 == 2 & u2 == 0)
  Clock1 : Clock
  UDP Send (Clock) : nvidiaSharedBlocks/UDP Send  remoteURL='255.255.255.255'  remotePort=48741  localURL='0.0.0.0'  localPortSource=Automatically determine  localPort=-1  sampletime=-1  blockPlatform=NVIDIA  separateLengthPort=0
      settings: LibrarySourceBlock=nvidiaNetworklib/UDP Send
  wires:
  Clock1/1 -> UDP Send (Clock)/1

== system GNC2026W/Time Sync./Change BLUE Behavior ==
  Action Port : ActionPort  ActionPortLabel=if(u1 == 3 & u2 == 0)
  Clock1 : Clock
  UDP Send (Clock) : nvidiaSharedBlocks/UDP Send  remoteURL='255.255.255.255'  remotePort=48742  localURL='0.0.0.0'  localPortSource=Automatically determine  localPort=-1  sampletime=-1  blockPlatform=NVIDIA  separateLengthPort=0
      settings: LibrarySourceBlock=nvidiaNetworklib/UDP Send
  wires:
  Clock1/1 -> UDP Send (Clock)/1

== system GNC2026W/Time Sync./Change RED Behavior ==
  Action Port : ActionPort  ActionPortLabel=if(u1 == 1 & u2 == 0)
  Clock1 : Clock
  UDP Send (Clock) : nvidiaSharedBlocks/UDP Send  remoteURL='255.255.255.255'  remotePort=48740  localURL='0.0.0.0'  localPortSource=Automatically determine  localPort=-1  sampletime=-1  blockPlatform=NVIDIA  separateLengthPort=0
      settings: LibrarySourceBlock=nvidiaNetworklib/UDP Send
  wires:
  Clock1/1 -> UDP Send (Clock)/1

== system GNC2026W/1 - Experiment Logic/Phase #2: Initial Position/Desired Joint Angles RED ==
  Constant1 : Constant  Value=pi/2
  Constant2 : Constant  Value=0
  Constant3 : Constant  Value=pi/2
  Mux : Mux  Inputs=3
  Target Array : Outport
  wires:
  Mux/1 -> Target Array/1
  Constant3/1 -> Mux/1
  Constant1/1 -> Mux/2
  Constant2/1 -> Mux/3

== system GNC2026W/1 - Experiment Logic/Phase #2: Initial Position/Desired Position BLACK ==
  Desired States (BLACK) : Constant  Value=init_states_BLACK  SampleTime=-1
  Target Array : Outport
  wires:
  Desired States (BLACK)/1 -> Target Array/1

== system GNC2026W/1 - Experiment Logic/Phase #2: Initial Position/Desired Position BLUE ==
  Desired States (BLUE) : Constant  Value=init_states_BLUE  SampleTime=-1
  Target Array : Outport
  wires:
  Desired States (BLUE)/1 -> Target Array/1

== system GNC2026W/1 - Experiment Logic/Phase #2: Initial Position/Desired Position RED ==
  Constant2 : Constant  Value=init_states_RED
  Target Array : Outport
  wires:
  Constant2/1 -> Target Array/1

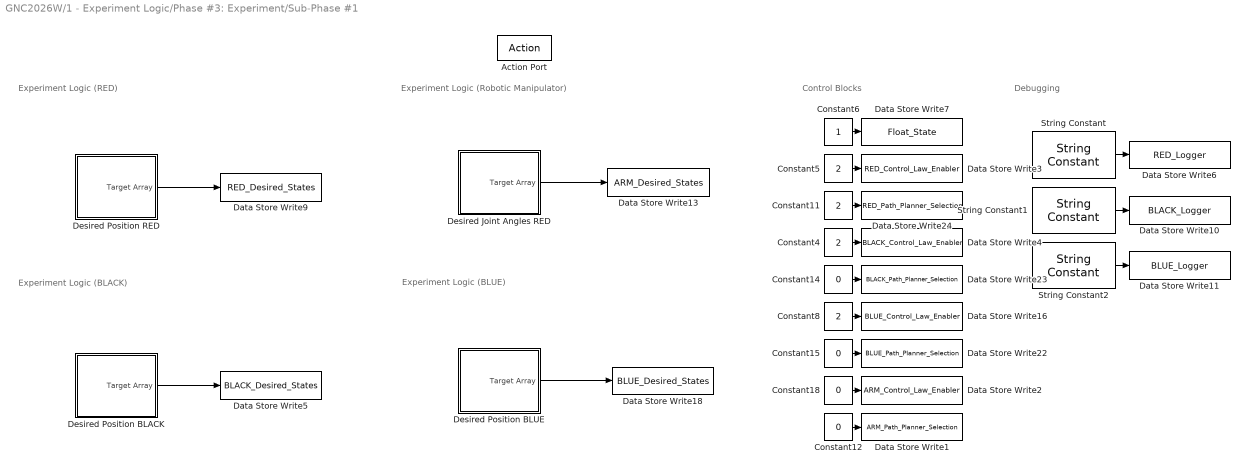
== system GNC2026W/1 - Experiment Logic/Phase #3: Experiment/Sub-Phase #1 ==
  note: Experiment Logic (BLUE)
  note: Experiment Logic (Robotic Manipulator)
  note: Experiment Logic (RED)
  note: Experiment Logic (BLACK)
  note: Control Blocks
  note: Debugging
  Action Port : ActionPort  ActionPortLabel=if(u1 < u2)
  Constant{4..5,8,11} (4 alike) : Constant  Value=2
  Constant{12,14..15,18} (4 alike) : Constant  Value=0
  Constant6 : Constant
  Data Store Write1 : DataStoreWrite  DataStoreName=ARM_Path_Planner_Selection  IndexOptions=Index vector (dialog)  Indices=1  OutputSizes=1
  Data Store Write10 : DataStoreWrite  DataStoreName=BLACK_Logger  IndexOptions=Index vector (dialog)  Indices=1  OutputSizes=1
  Data Store Write11 : DataStoreWrite  DataStoreName=BLUE_Logger  IndexOptions=Index vector (dialog)  Indices=1  OutputSizes=1
  Data Store Write13 : DataStoreWrite  DataStoreName=ARM_Desired_States  IndexOptions=Index vector (dialog)  Indices=1  OutputSizes=1
  Data Store Write16 : DataStoreWrite  DataStoreName=BLUE_Control_Law_Enabler  IndexOptions=Index vector (dialog)  Indices=1  OutputSizes=1
  Data Store Write18 : DataStoreWrite  DataStoreName=BLUE_Desired_States  IndexOptions=Index vector (dialog)  Indices=1  OutputSizes=1
  Data Store Write2 : DataStoreWrite  DataStoreName=ARM_Control_Law_Enabler  IndexOptions=Index vector (dialog)  Indices=1  OutputSizes=1
  Data Store Write22 : DataStoreWrite  DataStoreName=BLUE_Path_Planner_Selection  IndexOptions=Index vector (dialog)  Indices=1  OutputSizes=1
  Data Store Write23 : DataStoreWrite  DataStoreName=BLACK_Path_Planner_Selection  IndexOptions=Index vector (dialog)  Indices=1  OutputSizes=1
  Data Store Write24 : DataStoreWrite  DataStoreName=RED_Path_Planner_Selection  IndexOptions=Index vector (dialog)  Indices=1  OutputSizes=1
  Data Store Write3 : DataStoreWrite  DataStoreName=RED_Control_Law_Enabler  IndexOptions=Index vector (dialog)  Indices=1  OutputSizes=1
  Data Store Write4 : DataStoreWrite  DataStoreName=BLACK_Control_Law_Enabler  IndexOptions=Index vector (dialog)  Indices=1  OutputSizes=1
  Data Store Write5 : DataStoreWrite  DataStoreName=BLACK_Desired_States  IndexOptions=Index vector (dialog)  Indices=1  OutputSizes=1
  Data Store Write6 : DataStoreWrite  DataStoreName=RED_Logger  IndexOptions=Index vector (dialog)  Indices=1  OutputSizes=1
  Data Store Write7 : DataStoreWrite  DataStoreName=Float_State  IndexOptions=Index vector (dialog)  Indices=1  OutputSizes=1
  Data Store Write9 : DataStoreWrite  DataStoreName=RED_Desired_States  IndexOptions=Index vector (dialog)  Indices=1  OutputSizes=1
  Desired Joint Angles RED : Subsystem
  Desired Position BLACK : Subsystem
  Desired Position BLUE : Subsystem
  Desired Position RED : Subsystem
  String Constant : StringConstant  String="\"Chaser: Running Phase 3 Sub-Phase 1\""
  String Constant1 : StringConstant  String="\"Target: Running Phase 3 Sub-Phase 1\""
  String Constant2 : StringConstant  String="\"Obstacle: Running Phase 3 Sub-Phase 1\""
  wires:
  Desired Position BLACK/1(Target Array) -> Data Store Write5/1
  Desired Position BLUE/1(Target Array) -> Data Store Write18/1
  Desired Position RED/1(Target Array) -> Data Store Write9/1
  Desired Joint Angles RED/1(Target Array) -> Data Store Write13/1
  Constant12/1 -> Data Store Write1/1
  Constant18/1 -> Data Store Write2/1
  Constant6/1 -> Data Store Write7/1
  Constant15/1 -> Data Store Write22/1
  Constant14/1 -> Data Store Write23/1
  Constant5/1 -> Data Store Write3/1
  Constant11/1 -> Data Store Write24/1
  Constant8/1 -> Data Store Write16/1
  Constant4/1 -> Data Store Write4/1
  String Constant2/1 -> Data Store Write11/1
  String Constant1/1 -> Data Store Write10/1
  String Constant/1 -> Data Store Write6/1

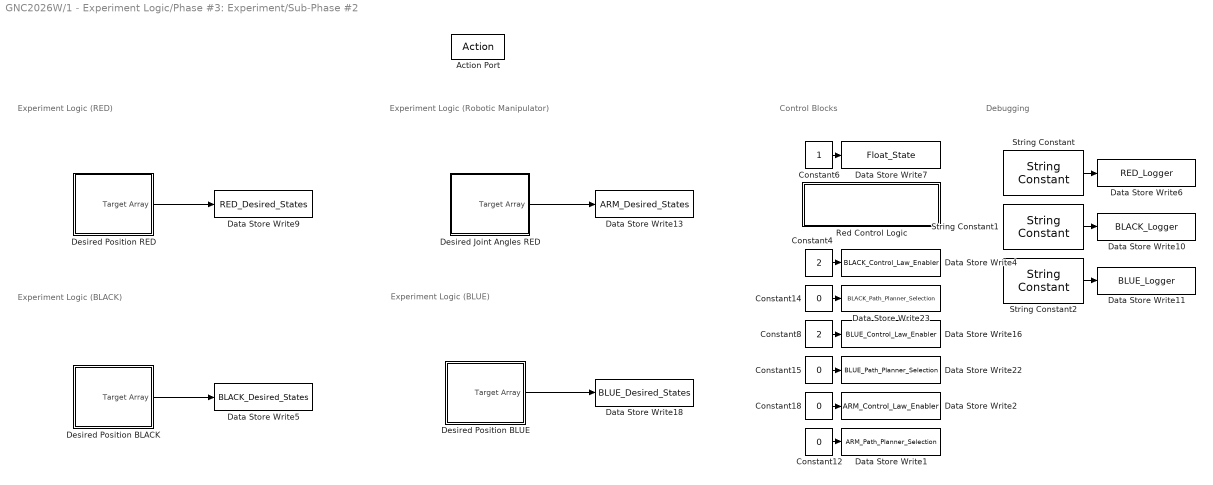
== system GNC2026W/1 - Experiment Logic/Phase #3: Experiment/Sub-Phase #2  ==
  note: Experiment Logic (BLACK)
  note: Experiment Logic (Robotic Manipulator)
  note: Experiment Logic (BLUE)
  note: Experiment Logic (RED)
  note: Control Blocks
  note: Debugging
  Action Port : ActionPort  ActionPortLabel=elseif((u1 < u3 & u1 >= u2))
  Constant{12,14..15,18} (4 alike) : Constant  Value=0
  Constant4 : Constant  Value=2
  Constant6 : Constant
  Constant8 : Constant  Value=2
  Data Store Write1 : DataStoreWrite  DataStoreName=ARM_Path_Planner_Selection  IndexOptions=Index vector (dialog)  Indices=1  OutputSizes=1
  Data Store Write10 : DataStoreWrite  DataStoreName=BLACK_Logger  IndexOptions=Index vector (dialog)  Indices=1  OutputSizes=1
  Data Store Write11 : DataStoreWrite  DataStoreName=BLUE_Logger  IndexOptions=Index vector (dialog)  Indices=1  OutputSizes=1
  Data Store Write13 : DataStoreWrite  DataStoreName=ARM_Desired_States  IndexOptions=Index vector (dialog)  Indices=1  OutputSizes=1
  Data Store Write16 : DataStoreWrite  DataStoreName=BLUE_Control_Law_Enabler  IndexOptions=Index vector (dialog)  Indices=1  OutputSizes=1
  Data Store Write18 : DataStoreWrite  DataStoreName=BLUE_Desired_States  IndexOptions=Index vector (dialog)  Indices=1  OutputSizes=1
  Data Store Write2 : DataStoreWrite  DataStoreName=ARM_Control_Law_Enabler  IndexOptions=Index vector (dialog)  Indices=1  OutputSizes=1
  Data Store Write22 : DataStoreWrite  DataStoreName=BLUE_Path_Planner_Selection  IndexOptions=Index vector (dialog)  Indices=1  OutputSizes=1
  Data Store Write23 : DataStoreWrite  DataStoreName=BLACK_Path_Planner_Selection  IndexOptions=Index vector (dialog)  Indices=1  OutputSizes=1
  Data Store Write4 : DataStoreWrite  DataStoreName=BLACK_Control_Law_Enabler  IndexOptions=Index vector (dialog)  Indices=1  OutputSizes=1
  Data Store Write5 : DataStoreWrite  DataStoreName=BLACK_Desired_States  IndexOptions=Index vector (dialog)  Indices=1  OutputSizes=1
  Data Store Write6 : DataStoreWrite  DataStoreName=RED_Logger  IndexOptions=Index vector (dialog)  Indices=1  OutputSizes=1
  Data Store Write7 : DataStoreWrite  DataStoreName=Float_State  IndexOptions=Index vector (dialog)  Indices=1  OutputSizes=1
  Data Store Write9 : DataStoreWrite  DataStoreName=RED_Desired_States  IndexOptions=Index vector (dialog)  Indices=1  OutputSizes=1
  Desired Joint Angles RED : Subsystem
  Desired Position BLACK : Subsystem
  Desired Position BLUE : Subsystem
  Desired Position RED : Subsystem
  Red Control Logic : Subsystem
  String Constant : StringConstant  String="\"Chaser: Running Phase 3 Sub-Phase 2\""
  String Constant1 : StringConstant  String="\"Target: Running Phase 3 Sub-Phase 2\""
  String Constant2 : StringConstant  String="\"Obstacle: Running Phase 3 Sub-Phase 2\""
  wires:
  Desired Position RED/1(Target Array) -> Data Store Write9/1
  Desired Position BLACK/1(Target Array) -> Data Store Write5/1
  Desired Position BLUE/1(Target Array) -> Data Store Write18/1
  Constant12/1 -> Data Store Write1/1
  Constant18/1 -> Data Store Write2/1
  Constant6/1 -> Data Store Write7/1
  Constant15/1 -> Data Store Write22/1
  Constant14/1 -> Data Store Write23/1
  Constant8/1 -> Data Store Write16/1
  Constant4/1 -> Data Store Write4/1
  Desired Joint Angles RED/1(Target Array) -> Data Store Write13/1
  String Constant1/1 -> Data Store Write10/1
  String Constant/1 -> Data Store Write6/1
  String Constant2/1 -> Data Store Write11/1
